simulink model "mfordmodel_v1"  (R2023a)
settings: Solver=ode45  StartTime=0.0  StopTime=10.0  RelTol=1e-3  EnableMultiTasking=on
undefined symbols (not defined in the file): ABV_RATIO_SW, AC_OFF_DLY, ACLOD, AUTO_TRNS_SW, BRAKE_DNDT_X, BZZRPM, BZZRPM_ALT, BZZTM, BZZTM_ALT, CMD_LITOFF, CMD_STABLE, CO_ST_ECT__A, COOL_BASE, DAS_BKDLY_A, DAS_CNT, DAS_CTDLY, DAS_LC_SW__A, DASCLP_5INH, DASCTL, DASMHYST, DASMPH, DEBYCP, DES_BASE, DPNEU_MUL, DSDRPM_DN_TC, DSDRPM_OFF, DSDRPM_UP_TC, EDF_DELAY, EDFHP, ETC_CL_TP, ETC_HP, GR_CM_CREEP, HCAM_ACT_CLP, HEDFHP, HEDFRPM, HICAM_PS, IAC_CAL_SW, IAC_ER_TM1, IAC_ER_TM2, IAC_ER_TM4, IAC_HI_LIM__A, IAC_ISFL_OBD, IAC_KAM_SW, IAC_LO_LIM__A, IAC_MON_TM, IAC_OT_REQ, IAC_RUN_TM, IAC_TP_OBD, IAC_TR_DAS, IAC_TST_DC, ID_DAS__A, ID_NOVS__A, IDVS_CH__A, IDVS_SL__A, IPSI_SW, IPSIDLY, IS_DRBASE__A, IS_DRBASE_A__A, IS_NUBASE__A, IS_NUBASE_A__A ... (+35)
libraries: simulink x2
(part 11 of 12)

== stateflow chart mfordmodel_v1/iac_v04_001_001/iac_executive/misc_calcs/TIMER_DT_in/Timer Control ==
  state TIMER_control
    state CHANGE_timer
      /* only one
      flag active */
      CHANGE_timer -> (junction 25) [order 1]
      (junction 26) -> (junction 25) [order 2]
      (junction 25) -> (junction 28) [order 1] : [incr_flag==1]
          | {
          | count_direction=1;
          | }
      (junction 25) -> (junction 28) [order 2] : [decr_flag==1]
          | {
          | count_direction= -1;
          | }
      (default) -> (junction 26)
      (junction 26) -> (junction 30) [order 1] : [reset_flag == 1]
          | {reset_flag = 0;}
      (junction 28) -> (junction 30) : {
          | do_delta_time;
          | do_timer;
          | }
    state HOLD_timer
      /* flags both
      active or both
      inactive */
      (default) -> (junction 27)
      (junction 27) -> (junction 29) : {
          | count_direction=0;
          | do_delta_time;
          | }
    (default) -> (junction 23)
    (junction 23) -> HOLD_timer [order 2]
    (junction 23) -> CHANGE_timer [order 1] : [incr_flag!=decr_flag]
    HOLD_timer -> (junction 27) [order 2]
    HOLD_timer -> CHANGE_timer [order 1] : [incr_flag!=decr_flag]
    CHANGE_timer -> HOLD_timer [order 1] : [incr_flag==decr_flag]
  (default) -> (junction 24)
  (junction 24) -> TIMER_control [order 2]
  (junction 24) -> TIMER_control [order 1] : trig_reset
      | {
      | reset_flag=1;
      | do_delta_time;
      | do_timer;
      | }
  TIMER_control -> TIMER_control : trig_reset
      | {
      | reset_flag=1;
      | do_delta_time;
      | do_timer;
      | }
  data: count_direction output int16; incr_flag input boolean; decr_flag input boolean; reset_flag output boolean [0..1]
  events: do_delta_time output FUNCTION_CALL_EVENT; do_timer output FUNCTION_CALL_EVENT; trig_timer input FUNCTION_CALL_EVENT; trig_reset input FUNCTION_CALL_EVENT

== stateflow chart mfordmodel_v1/iac_v04_001_001/activate_desired_rpm/rpm_adders_fans_and_pw_steer/rpm_adders_fans_pw_steer_ctl ==
  (default) -> (junction 6) : trig_rpm_adders_fans_pw_steer
  (junction 6) -> (junction 7) [order 2] : { is_hedf_rpm = 0.0; }
  (junction 6) -> (junction 7) [order 1] : [   (HEDFHP == 1)...
      |  && (hsf_flg == 1) ]
      | { is_hedf_rpm =HEDFRPM; }
  (junction 7) -> (junction 8) [order 1] : [ powsfg == 1 ]
      | { is_ps_rpm = PS_RPM; }
  (junction 7) -> (junction 8) [order 2] : { is_ps_rpm = 0.0; }
  data: HEDFHP parameter boolean size=1; hsf_flg input boolean size=1; is_hedf_rpm output double size=1; powsfg input boolean size=1; is_ps_rpm output double size=1; PS_RPM parameter double size=1; HEDFRPM parameter double size=1
  events: trig_rpm_adders_fans_pw_steer input FUNCTION_CALL_EVENT

== stateflow chart mfordmodel_v1/iac_v04_001_001/iac_executive/runup_flag_timer/TIMER_DT_in/Timer Control ==
  state TIMER_control
    state CHANGE_timer
      /* only one
      flag active */
      CHANGE_timer -> (junction 25) [order 1]
      (junction 26) -> (junction 25) [order 2]
      (junction 25) -> (junction 28) [order 1] : [incr_flag==1]
          | {
          | count_direction=1;
          | }
      (junction 25) -> (junction 28) [order 2] : [decr_flag==1]
          | {
          | count_direction= -1;
          | }
      (default) -> (junction 26)
      (junction 26) -> (junction 30) [order 1] : [reset_flag == 1]
          | {reset_flag = 0;}
      (junction 28) -> (junction 30) : {
          | do_delta_time;
          | do_timer;
          | }
    state HOLD_timer
      /* flags both
      active or both
      inactive */
      (default) -> (junction 27)
      (junction 27) -> (junction 29) : {
          | count_direction=0;
          | do_delta_time;
          | }
    (default) -> (junction 23)
    (junction 23) -> HOLD_timer [order 2]
    (junction 23) -> CHANGE_timer [order 1] : [incr_flag!=decr_flag]
    HOLD_timer -> (junction 27) [order 2]
    HOLD_timer -> CHANGE_timer [order 1] : [incr_flag!=decr_flag]
    CHANGE_timer -> HOLD_timer [order 1] : [incr_flag==decr_flag]
  (default) -> (junction 24)
  (junction 24) -> TIMER_control [order 2]
  (junction 24) -> TIMER_control [order 1] : trig_reset
      | {
      | reset_flag=1;
      | do_delta_time;
      | do_timer;
      | }
  TIMER_control -> TIMER_control : trig_reset
      | {
      | reset_flag=1;
      | do_delta_time;
      | do_timer;
      | }
  data: count_direction output int16; incr_flag input boolean; decr_flag input boolean; reset_flag output boolean [0..1]
  events: do_delta_time output FUNCTION_CALL_EVENT; do_timer output FUNCTION_CALL_EVENT; trig_timer input FUNCTION_CALL_EVENT; trig_reset input FUNCTION_CALL_EVENT

== stateflow chart mfordmodel_v1/iac_v04_001_001/normal_mode/activate_feedforward/ac_ppm_tmr/Timer Control ==
  state TIMER_control
    state CHANGE_timer
      /* only one
      flag active */
      CHANGE_timer -> (junction 23) [order 1]
      (default) -> (junction 23)
      (junction 23) -> (junction 25) [order 1] : [incr_flag==1]
          | {
          | count_direction=1;
          | }
      (junction 23) -> (junction 25) [order 2] : [decr_flag==1]
          | {
          | count_direction=(-1);
          | }
      (junction 25) -> (junction 27) : {
          | do_delta_time;
          | do_timer;
          | }
    state HOLD_timer
      /* flags both
      active or both
      inactive */
      (default) -> (junction 24)
      (junction 24) -> (junction 26) : {
          | count_direction=0;
          | do_delta_time;
          | }
    (default) -> (junction 21) : {
        | reset_flag=0;
        | }
    (junction 21) -> HOLD_timer [order 2]
    (junction 21) -> CHANGE_timer [order 1] : [incr_flag!=decr_flag]
    HOLD_timer -> (junction 24) [order 2]
    HOLD_timer -> CHANGE_timer [order 1] : [incr_flag!=decr_flag]
    CHANGE_timer -> HOLD_timer [order 1] : [incr_flag==decr_flag]
  (default) -> (junction 22)
  (junction 22) -> TIMER_control [order 2]
  (junction 22) -> TIMER_control [order 1] : trig_reset
      | {
      | reset_flag=1;
      | do_delta_time;
      | do_timer;
      | }
  TIMER_control -> TIMER_control : trig_reset
      | {
      | reset_flag=1;
      | do_delta_time;
      | do_timer;
      | }
  data: count_direction output int16; incr_flag input boolean; decr_flag input boolean; reset_flag output boolean [0..1]
  events: do_delta_time output FUNCTION_CALL_EVENT; do_timer output FUNCTION_CALL_EVENT; trig_timer input FUNCTION_CALL_EVENT; trig_reset input FUNCTION_CALL_EVENT

== stateflow chart mfordmodel_v1/iac_v04_001_001/normal_mode/activate_kam/iac_kam_tmr/Timer Control ==
  state TIMER_control
    state CHANGE_timer
      /* only one
      flag active */
      CHANGE_timer -> (junction 23) [order 1]
      (default) -> (junction 23)
      (junction 23) -> (junction 25) [order 1] : [incr_flag==1]
          | {
          | count_direction=1;
          | }
      (junction 23) -> (junction 25) [order 2] : [decr_flag==1]
          | {
          | count_direction=(-1);
          | }
      (junction 25) -> (junction 27) : {
          | do_delta_time;
          | do_timer;
          | }
    state HOLD_timer
      /* flags both
      active or both
      inactive */
      (default) -> (junction 24)
      (junction 24) -> (junction 26) : {
          | count_direction=0;
          | do_delta_time;
          | }
    (default) -> (junction 21) : {
        | reset_flag=0;
        | }
    (junction 21) -> HOLD_timer [order 2]
    (junction 21) -> CHANGE_timer [order 1] : [incr_flag!=decr_flag]
    HOLD_timer -> (junction 24) [order 2]
    HOLD_timer -> CHANGE_timer [order 1] : [incr_flag!=decr_flag]
    CHANGE_timer -> HOLD_timer [order 1] : [incr_flag==decr_flag]
  (default) -> (junction 22)
  (junction 22) -> TIMER_control [order 2]
  (junction 22) -> TIMER_control [order 1] : trig_reset
      | {
      | reset_flag=1;
      | do_delta_time;
      | do_timer;
      | }
  TIMER_control -> TIMER_control : trig_reset
      | {
      | reset_flag=1;
      | do_delta_time;
      | do_timer;
      | }
  data: count_direction output int16; incr_flag input boolean; decr_flag input boolean; reset_flag output boolean [0..1]
  events: do_delta_time output FUNCTION_CALL_EVENT; do_timer output FUNCTION_CALL_EVENT; trig_timer input FUNCTION_CALL_EVENT; trig_reset input FUNCTION_CALL_EVENT

== stateflow chart mfordmodel_v1/iac_v04_001_001/normal_mode/activate_normal_mode/normal_mode_fault_codes/iac_er_tmr1/Timer Control ==
  state TIMER_control
    state CHANGE_timer
      /* only one
      flag active */
      CHANGE_timer -> (junction 23) [order 1]
      (default) -> (junction 23)
      (junction 23) -> (junction 25) [order 1] : [incr_flag==1]
          | {
          | count_direction=1;
          | }
      (junction 23) -> (junction 25) [order 2] : [decr_flag==1]
          | {
          | count_direction=(-1);
          | }
      (junction 25) -> (junction 27) : {
          | do_delta_time;
          | do_timer;
          | }
    state HOLD_timer
      /* flags both
      active or both
      inactive */
      (default) -> (junction 24)
      (junction 24) -> (junction 26) : {
          | count_direction=0;
          | do_delta_time;
          | }
    (default) -> (junction 21) : {
        | reset_flag=0;
        | }
    (junction 21) -> HOLD_timer [order 2]
    (junction 21) -> CHANGE_timer [order 1] : [incr_flag!=decr_flag]
    HOLD_timer -> (junction 24) [order 2]
    HOLD_timer -> CHANGE_timer [order 1] : [incr_flag!=decr_flag]
    CHANGE_timer -> HOLD_timer [order 1] : [incr_flag==decr_flag]
  (default) -> (junction 22)
  (junction 22) -> TIMER_control [order 2]
  (junction 22) -> TIMER_control [order 1] : trig_reset
      | {
      | reset_flag=1;
      | do_delta_time;
      | do_timer;
      | }
  TIMER_control -> TIMER_control : trig_reset
      | {
      | reset_flag=1;
      | do_delta_time;
      | do_timer;
      | }
  data: count_direction output int16; incr_flag input boolean; decr_flag input boolean; reset_flag output boolean [0..1]
  events: do_delta_time output FUNCTION_CALL_EVENT; do_timer output FUNCTION_CALL_EVENT; trig_timer input FUNCTION_CALL_EVENT; trig_reset input FUNCTION_CALL_EVENT

== stateflow chart mfordmodel_v1/iac_v04_001_001/normal_mode/activate_normal_mode/normal_mode_fault_codes/iac_er_tmr2/Timer Control ==
  state TIMER_control
    state CHANGE_timer
      /* only one
      flag active */
      CHANGE_timer -> (junction 23) [order 1]
      (default) -> (junction 23)
      (junction 23) -> (junction 25) [order 1] : [incr_flag==1]
          | {
          | count_direction=1;
          | }
      (junction 23) -> (junction 25) [order 2] : [decr_flag==1]
          | {
          | count_direction=(-1);
          | }
      (junction 25) -> (junction 27) : {
          | do_delta_time;
          | do_timer;
          | }
    state HOLD_timer
      /* flags both
      active or both
      inactive */
      (default) -> (junction 24)
      (junction 24) -> (junction 26) : {
          | count_direction=0;
          | do_delta_time;
          | }
    (default) -> (junction 21) : {
        | reset_flag=0;
        | }
    (junction 21) -> HOLD_timer [order 2]
    (junction 21) -> CHANGE_timer [order 1] : [incr_flag!=decr_flag]
    HOLD_timer -> (junction 24) [order 2]
    HOLD_timer -> CHANGE_timer [order 1] : [incr_flag!=decr_flag]
    CHANGE_timer -> HOLD_timer [order 1] : [incr_flag==decr_flag]
  (default) -> (junction 22)
  (junction 22) -> TIMER_control [order 2]
  (junction 22) -> TIMER_control [order 1] : trig_reset
      | {
      | reset_flag=1;
      | do_delta_time;
      | do_timer;
      | }
  TIMER_control -> TIMER_control : trig_reset
      | {
      | reset_flag=1;
      | do_delta_time;
      | do_timer;
      | }
  data: count_direction output int16; incr_flag input boolean; decr_flag input boolean; reset_flag output boolean [0..1]
  events: do_delta_time output FUNCTION_CALL_EVENT; do_timer output FUNCTION_CALL_EVENT; trig_timer input FUNCTION_CALL_EVENT; trig_reset input FUNCTION_CALL_EVENT

== stateflow chart mfordmodel_v1/iac_v04_001_001/normal_mode/activate_normal_mode/normal_mode_fault_codes/iac_mon_tmr/Timer Control ==
  state TIMER_control
    state CHANGE_timer
      /* only one
      flag active */
      CHANGE_timer -> (junction 23) [order 1]
      (default) -> (junction 23)
      (junction 23) -> (junction 25) [order 1] : [incr_flag==1]
          | {
          | count_direction=1;
          | }
      (junction 23) -> (junction 25) [order 2] : [decr_flag==1]
          | {
          | count_direction=(-1);
          | }
      (junction 25) -> (junction 27) : {
          | do_delta_time;
          | do_timer;
          | }
    state HOLD_timer
      /* flags both
      active or both
      inactive */
      (default) -> (junction 24)
      (junction 24) -> (junction 26) : {
          | count_direction=0;
          | do_delta_time;
          | }
    (default) -> (junction 21) : {
        | reset_flag=0;
        | }
    (junction 21) -> HOLD_timer [order 2]
    (junction 21) -> CHANGE_timer [order 1] : [incr_flag!=decr_flag]
    HOLD_timer -> (junction 24) [order 2]
    HOLD_timer -> CHANGE_timer [order 1] : [incr_flag!=decr_flag]
    CHANGE_timer -> HOLD_timer [order 1] : [incr_flag==decr_flag]
  (default) -> (junction 22)
  (junction 22) -> TIMER_control [order 2]
  (junction 22) -> TIMER_control [order 1] : trig_reset
      | {
      | reset_flag=1;
      | do_delta_time;
      | do_timer;
      | }
  TIMER_control -> TIMER_control : trig_reset
      | {
      | reset_flag=1;
      | do_delta_time;
      | do_timer;
      | }
  data: count_direction output int16; incr_flag input boolean; decr_flag input boolean; reset_flag output boolean [0..1]
  events: do_delta_time output FUNCTION_CALL_EVENT; do_timer output FUNCTION_CALL_EVENT; trig_timer input FUNCTION_CALL_EVENT; trig_reset input FUNCTION_CALL_EVENT

== stateflow chart mfordmodel_v1/iac_v04_001_001/normal_mode/activate_normal_mode/normal_mode_fault_codes/type1_fault_code/fault code_ctl ==
  state clear [parallel]
    settings: executionOrder=1
    clear -> (junction 9) : clear_malf
    (default) -> (junction 9) : clear_malf
    (junction 9) -> (junction 12) : {pxxxmalf = 0;}
  state malf [parallel]
    settings: executionOrder=2
    malf -> (junction 10) : malfunction
    (default) -> (junction 10) : malfunction
    (junction 10) -> (junction 11) : {pxxxmalf = 1;}
  data: pxxxmalf output double
  events: malfunction input FUNCTION_CALL_EVENT; clear_malf input FUNCTION_CALL_EVENT

== stateflow chart mfordmodel_v1/iac_v04_001_001/normal_mode/activate_normal_mode/normal_mode_fault_codes/type1_fault_code1/fault code_ctl ==
  state clear [parallel]
    settings: executionOrder=1
    clear -> (junction 9) : clear_malf
    (default) -> (junction 9) : clear_malf
    (junction 9) -> (junction 12) : {pxxxmalf = 0;}
  state malf [parallel]
    settings: executionOrder=2
    malf -> (junction 10) : malfunction
    (default) -> (junction 10) : malfunction
    (junction 10) -> (junction 11) : {pxxxmalf = 1;}
  data: pxxxmalf output double
  events: malfunction input FUNCTION_CALL_EVENT; clear_malf input FUNCTION_CALL_EVENT

== stateflow chart mfordmodel_v1/iac_v04_001_001/normal_mode/iscflg_module/dashpot/TIMER/Timer Control ==
  state TIMER_control
    state CHANGE_timer
      /* only one
      flag active */
      CHANGE_timer -> (junction 23) [order 1]
      (default) -> (junction 23)
      (junction 23) -> (junction 25) [order 1] : [incr_flag==1]
          | {
          | count_direction=1;
          | }
      (junction 23) -> (junction 25) [order 2] : [decr_flag==1]
          | {
          | count_direction=(-1);
          | }
      (junction 25) -> (junction 27) : {
          | do_delta_time;
          | do_timer;
          | }
    state HOLD_timer
      /* flags both
      active or both
      inactive */
      (default) -> (junction 24)
      (junction 24) -> (junction 26) : {
          | count_direction=0;
          | do_delta_time;
          | }
    (default) -> (junction 21) : {
        | reset_flag=0;
        | }
    (junction 21) -> HOLD_timer [order 2]
    (junction 21) -> CHANGE_timer [order 1] : [incr_flag!=decr_flag]
    HOLD_timer -> (junction 24) [order 2]
    HOLD_timer -> CHANGE_timer [order 1] : [incr_flag!=decr_flag]
    CHANGE_timer -> HOLD_timer [order 1] : [incr_flag==decr_flag]
  (default) -> (junction 22)
  (junction 22) -> TIMER_control [order 2]
  (junction 22) -> TIMER_control [order 1] : trig_reset
      | {
      | reset_flag=1;
      | do_delta_time;
      | do_timer;
      | }
  TIMER_control -> TIMER_control : trig_reset
      | {
      | reset_flag=1;
      | do_delta_time;
      | do_timer;
      | }
  data: count_direction output int16; incr_flag input boolean; decr_flag input boolean; reset_flag output boolean [0..1]
  events: do_delta_time output FUNCTION_CALL_EVENT; do_timer output FUNCTION_CALL_EVENT; trig_timer input FUNCTION_CALL_EVENT; trig_reset input FUNCTION_CALL_EVENT

== stateflow chart mfordmodel_v1/iac_v04_001_001/normal_mode/iscflg_module/iscflg_modes/1/Timer Control ==
  state TIMER_control
    state CHANGE_timer
      /* only one
      flag active */
      CHANGE_timer -> (junction 23) [order 1]
      (default) -> (junction 23)
      (junction 23) -> (junction 25) [order 1] : [incr_flag==1]
          | {
          | count_direction=1;
          | }
      (junction 23) -> (junction 25) [order 2] : [decr_flag==1]
          | {
          | count_direction=(-1);
          | }
      (junction 25) -> (junction 27) : {
          | do_delta_time;
          | do_timer;
          | }
    state HOLD_timer
      /* flags both
      active or both
      inactive */
      (default) -> (junction 24)
      (junction 24) -> (junction 26) : {
          | count_direction=0;
          | do_delta_time;
          | }
    (default) -> (junction 21) : {
        | reset_flag=0;
        | }
    (junction 21) -> HOLD_timer [order 2]
    (junction 21) -> CHANGE_timer [order 1] : [incr_flag!=decr_flag]
    HOLD_timer -> (junction 24) [order 2]
    HOLD_timer -> CHANGE_timer [order 1] : [incr_flag!=decr_flag]
    CHANGE_timer -> HOLD_timer [order 1] : [incr_flag==decr_flag]
  (default) -> (junction 22)
  (junction 22) -> TIMER_control [order 2]
  (junction 22) -> TIMER_control [order 1] : trig_reset
      | {
      | reset_flag=1;
      | do_delta_time;
      | do_timer;
      | }
  TIMER_control -> TIMER_control : trig_reset
      | {
      | reset_flag=1;
      | do_delta_time;
      | do_timer;
      | }
  data: count_direction output int16; incr_flag input boolean; decr_flag input boolean; reset_flag output boolean [0..1]
  events: do_delta_time output FUNCTION_CALL_EVENT; do_timer output FUNCTION_CALL_EVENT; trig_timer input FUNCTION_CALL_EVENT; trig_reset input FUNCTION_CALL_EVENT

== stateflow chart mfordmodel_v1/iac_v04_001_001/iac_executive/misc_calcs/misc_calcs_ctl ==
  (default) -> (junction 9) : {
      |  trig_osc_response_logic;
      | }
  (junction 9) -> (junction 11) [order 2] : /* gear5tmr_update */
  (junction 9) -> (junction 10) [order 1] : [ TRLOAD > 3 ]
  (junction 10) -> (junction 11) [order 1] : [ gr_cm != 5 ]
      | {
      |   gear5th = 0;
      |   trig_rst_gear5tmr;
      | }
  (junction 10) -> (junction 11) [order 2] : {
      |  gear5th = 1;
      |  trig_incr_gear5tmr;
      | }
  (junction 11) -> (junction 12) [order 1] : /* dndt_das_update() */
      |
      | [  (eng_stalled == 1)...
      |  || ( apt >= 0) ]
      | {
      | ml_dndt_sw = 1;
      | }
  (junction 11) -> (junction 12) [order 2] : {
      |  ml_dndt_sw = 2;
      | }
  (junction 12) -> (junction 13) : {
      | do_dndt_calc;
      | }
  data: TRLOAD parameter uint8 size=1; gear5th output boolean size=1; ml_dndt_sw output uint8 size=1 =1; eng_stalled input boolean size=1; gr_cm input uint8 size=1; apt input int8 size=1
  events: trig_incr_gear5tmr output FUNCTION_CALL_EVENT; trig_rst_gear5tmr output FUNCTION_CALL_EVENT; trig_misc_calcs input FUNCTION_CALL_EVENT; do_dndt_calc output FUNCTION_CALL_EVENT; trig_osc_response_logic output FUNCTION_CALL_EVENT

== stateflow chart mfordmodel_v1/iac_v04_001_001/normal_mode/iscflg_module/iscflg_modes/2/Timer Control ==
  state TIMER_control
    state CHANGE_timer
      /* only one
      flag active */
      CHANGE_timer -> (junction 23) [order 1]
      (default) -> (junction 23)
      (junction 23) -> (junction 25) [order 1] : [incr_flag==1]
          | {
          | count_direction=1;
          | }
      (junction 23) -> (junction 25) [order 2] : [decr_flag==1]
          | {
          | count_direction=(-1);
          | }
      (junction 25) -> (junction 27) : {
          | do_delta_time;
          | do_timer;
          | }
    state HOLD_timer
      /* flags both
      active or both
      inactive */
      (default) -> (junction 24)
      (junction 24) -> (junction 26) : {
          | count_direction=0;
          | do_delta_time;
          | }
    (default) -> (junction 21) : {
        | reset_flag=0;
        | }
    (junction 21) -> HOLD_timer [order 2]
    (junction 21) -> CHANGE_timer [order 1] : [incr_flag!=decr_flag]
    HOLD_timer -> (junction 24) [order 2]
    HOLD_timer -> CHANGE_timer [order 1] : [incr_flag!=decr_flag]
    CHANGE_timer -> HOLD_timer [order 1] : [incr_flag==decr_flag]
  (default) -> (junction 22)
  (junction 22) -> TIMER_control [order 2]
  (junction 22) -> TIMER_control [order 1] : trig_reset
      | {
      | reset_flag=1;
      | do_delta_time;
      | do_timer;
      | }
  TIMER_control -> TIMER_control : trig_reset
      | {
      | reset_flag=1;
      | do_delta_time;
      | do_timer;
      | }
  data: count_direction output int16; incr_flag input boolean; decr_flag input boolean; reset_flag output boolean [0..1]
  events: do_delta_time output FUNCTION_CALL_EVENT; do_timer output FUNCTION_CALL_EVENT; trig_timer input FUNCTION_CALL_EVENT; trig_reset input FUNCTION_CALL_EVENT

== stateflow chart mfordmodel_v1/iac_v04_001_001/normal_mode/activate_feedforward/activate_feedforward_ctl ==
  state ac_ppm [parallel]
    settings: executionOrder=1
    ac_ppm -> (junction 43) : trig
    (default) -> (junction 43) : trig
    (junction 43) -> (junction 47) [order 1] : [ ac_ppm_rqst == 0 ]
        | {
        | ml_ac_sw = 3 ;
        | }
    (junction 43) -> (junction 45) [order 2]
    (junction 45) -> (junction 47) [order 2] : {
        | ml_ac_sw = 1 ;
        | }
    (junction 45) -> (junction 47) [order 1] : [ ac_cycle_flg == 0 ]
        | {
        | ml_ac_sw = 2 ;
        | }
    (junction 47) -> (junction 49) [order 2] : {
        | trig_ac_ppm_tmr_update;
        | }
    (junction 47) -> (junction 49) [order 1] : [ ac_ppm_rqst == 0 ]
        | {
        | trig_ac_ppm_tmr_reset;
        | }
  state fan_ppm_calc [parallel]
    settings: executionOrder=2
    fan_ppm_calc -> (junction 42) : trig
    (junction 42) -> (junction 48) [order 1] : [ (EDFHP == 1)...
        |  && ( VSFOP_HP== 0 )...
        |  && (VFD_HP == 0 )...
        |  && ( lsf_rqst == 1 )...
        |  && ( fantmr >= EDF_DELAY) ]
        | {
        | ml_fan_sw = 1;
        | }
    (default) -> (junction 42) : trig
    (junction 42) -> (junction 44) [order 2]
    (junction 44) -> (junction 48) [order 1] : [ VSFOP_HP == 1 ]
        | {
        | ml_fan_sw = 2;
        | }
    (junction 44) -> (junction 46) [order 2]
    (junction 46) -> (junction 48) [order 2] : {
        | ml_fan_sw = 4;
        | }
    (junction 46) -> (junction 48) [order 1] : [ VFD_HP == 1 ]
        | {
        | ml_fan_sw = 3;
        | }
  state base_ppm [parallel]
    settings: executionOrder=3
    base_ppm -> (junction 50) : trig
    (default) -> (junction 50) : trig
    (junction 50) -> (junction 52) [order 1] : [ (AUTO_TRNS_SW == 0 )...
        |  || ( dndsup == 0 ) ]
        | {
        | ml_base_sw = 1  ;
        | }
    (junction 50) -> (junction 52) [order 2] : {
        | ml_base_sw = 2 ;
        | }
    (junction 52) -> (junction 55) [order 2] : {
        | ml_trans_sw = 2 ;
        | }
    (junction 52) -> (junction 55) [order 1] : [  ( idle_ppm <= DASCTL )...
        |  && (      ( pdl != PARK)...
        |          && (pdl != NEUTRAL) )...
        |  && ( apt == CLOSED_THROTTLE )...
        |  && ( ect > VSEECT )...
        |  && ( DES_BASE == 1 )...
        |  && ( vspd > MINMPH )...
        |  && ( gr_cm >= GR_CM_CREEP ) ]
        | {
        | ml_trans_sw = 1;
        | }
  state power_steering_ppm [parallel]
    settings: executionOrder=4
    power_steering_ppm -> (junction 51) : trig
    (default) -> (junction 51) : trig
    (junction 51) -> (junction 53) [order 1] : [  (powsfg == 1)...
        |  && ( PSPSHP == 1)...
        |  && ( hicam <= HICAM_PS) ]
    (junction 51) -> (junction 54) [order 2] : {
        | ml_ps_sw = 3;
        | }
    (junction 53) -> (junction 54) [order 2] : {
        | ml_ps_sw = 2 ;
        | }
    (junction 53) -> (junction 54) [order 1] : [ vspd < PS_VS ]
        | {
        | ml_ps_sw = 1 ;
        | }
  state fail_safe_cooling_ppm [parallel]
    settings: executionOrder=5
    fail_safe_cooling_ppm -> (junction 56) : trig
    (default) -> (junction 56) : trig
    (junction 56) -> (junction 58) [order 2] : {
        | ml_fsc_sw = 2 ;
        | }
    (junction 56) -> (junction 58) [order 1] : [ cool_flg == 1 ]
        | {
        | ml_fsc_sw = 1 ;
        | }
  state desmaf_pre_calcs [parallel]
    /* Must be lowest priority parallel state */
    settings: executionOrder=6
    desmaf_pre_calcs -> (junction 57) : trig_activate_feedforward
    (default) -> (junction 57) : trig_activate_feedforward
    (junction 57) -> (junction 59) : {
        | ac_ppm.trig;
        | fail_safe_cooling_ppm.trig;
        | fan_ppm_calc.trig;
        | base_ppm.trig;
        | power_steering_ppm.trig;
        | do_desmaf_pre_calc;
        | }
  data: dndsup input boolean size=1; ect input single size=1; idle_ppm input single size=1; pdl input uint8 size=1; apt input int8 size=1; vspd input single size=1; gr_cm input uint8 size=1; AUTO_TRNS_SW parameter uint8 size=1; DASCTL parameter single size=1; MINMPH parameter single size=1; VSEECT parameter single size=1; DES_BASE parameter single size=1; ac_cycle_flg input boolean size=1; ac_ppm_rqst input boolean size=1; ml_ac_sw output uint8 size=1; PS_VS parameter single size=1; PSPSHP parameter boolean size=1; powsfg input boolean size=1; cool_flg input boolean size=1; ml_ps_sw output uint8 size=1; ml_fsc_sw output uint8 size=1; ml_base_sw output uint8 size=1; ml_trans_sw output uint8 size=1; hicam input single size=1; HICAM_PS parameter single size=1; AUTOMATIC4 constant uint8 size=1 =4; CLOSED_THROTTLE constant int8 size=1 =-1; ml_fan_sw output int8 size=1 =3; VSFOP_HP parameter boolean size=1; EDFHP parameter boolean size=1; lsf_rqst input boolean size=1; EDF_DELAY parameter single size=1; fantmr input single size=1; VFD_HP parameter single size=1; GR_CM_CREEP parameter uint8 size=1; PARK constant uint8 size=1 =70; NEUTRAL constant uint8 size=1 =50
  events: trig local EITHER_EDGE_EVENT; trig local EITHER_EDGE_EVENT; trig local EITHER_EDGE_EVENT; trig local EITHER_EDGE_EVENT; trig local EITHER_EDGE_EVENT; trig_activate_feedforward input FUNCTION_CALL_EVENT; do_desmaf_pre_calc output FUNCTION_CALL_EVENT; trig_ac_ppm_tmr_update output FUNCTION_CALL_EVENT; trig_ac_ppm_tmr_reset output FUNCTION_CALL_EVENT

== stateflow chart mfordmodel_v1/iac_v04_001_001/normal_mode/iscflg_module/dashpot/activate_daspot_mode_ctl ==
  (default) -> (junction 20) : { trig_dec_das_delay; }
  (junction 20) -> (junction 21) [order 1] : /* no_decel_counter() */
      | [ ( gear5th == 0) ||...
      |   ( cttmr <= DAS_CTDLY) ]
  (junction 21) -> (junction 26) : { das_ctr = 0; }
  (junction 20) -> (junction 22) [order 2]
  (junction 22) -> (junction 23) [order 1] : [ (gear5th == 1) &&...
      |   ( cttmr > DAS_CTDLY) &&...
      |   ( dndt_das > DAS_DNDT_X) &&...
      |   ( das_ctr < 255 ) ]
  (junction 23) -> (junction 25) : { das_ctr = das_ctr + 1; }
  (junction 22) -> (junction 24) [order 2]
  (junction 25) -> (junction 24)
  (junction 26) -> (junction 25)
  (junction 24) -> (junction 27) : { trig_daspot_shift_trans_calc; }
  (junction 27) -> (junction 28) [order 1] : /* base_dashpot_calculation() */
      | [ (das_delay__A > 0.0)...
      |  && (das_ppm__A > 0.0) ]
  (junction 28) -> (junction 32) : { ml_idle_ppm_sw = 1; }
  (junction 27) -> (junction 29) [order 2]
  (junction 29) -> (junction 30) [order 1] : [ (flg_crv_lk == 1)...
      |  && (DAS_LC_SW__A == 1) ]
  (junction 30) -> (junction 33) : { ml_idle_ppm_sw = 2; }
  (junction 29) -> (junction 31) [order 2] : { ml_idle_ppm_sw = 3; }
  (junction 33) -> (junction 31)
  (junction 32) -> (junction 33)
  (junction 31) -> (junction 34) : { do_daspot_calc;
      |   trig_das_min_clip_daspot; }
  data: ml_idle_ppm_sw output uint8 size=1; das_delay__A input double size=1; das_ppm__A input double size=1; gear5th input boolean size=1; cttmr input single size=1; DAS_CTDLY parameter single size=1; DAS_DNDT_X constant single size=1; das_ctr output uint8 size=1; dndt_das input single size=1; ndsflg input boolean size=1; ptctfg input boolean size=1; TRLOAD parameter uint8 size=1; NRATCH_OFF constant boolean size=1; DAS_LC_SW__A constant boolean size=1; flg_crv_lk input boolean size=1; engine_speed input single size=1; CLOSED_THROTTLE constant int8 size=1 =-1; apt input int8 size=1
  events: trig_activate_daspot_mode input FUNCTION_CALL_EVENT; do_daspot_calc output FUNCTION_CALL_EVENT; trig_das_min_clip_daspot output FUNCTION_CALL_EVENT; trig_dec_das_delay output FUNCTION_CALL_EVENT; trig_daspot_shift_trans_calc output FUNCTION_CALL_EVENT

== stateflow chart mfordmodel_v1/iac_v04_001_001/normal_mode/iscflg_module/das_min_clip/das_min_clip_ctl ==
  state min_clip_calc [parallel]
    settings: executionOrder=1
    (default) -> (junction 88) : trig
    min_clip_calc -> (junction 88) : trig
    (junction 88) -> (junction 89) [order 1] : [ (dndsup == 0) && (TRLOAD > 3) ]
    (junction 89) -> (junction 91)
    (junction 88) -> (junction 90) [order 2]
    (junction 90) -> (junction 91) [order 1] : [ (DASCLP_5INH == 1) && (apt >= 0) && (gear5th == 1) && (flg_dasclp5 == 0) ]
    (junction 91) -> (junction 93)
    (junction 90) -> (junction 92) [order 2]
    (junction 92) -> (junction 93) [order 1] : [ (gear5tmr > DAS_BKDLY_A) && (dndt_das < BRAKE_DNDT_X) ]
    (junction 93) -> (junction 95)
    (junction 92) -> (junction 94) [order 2]
    (junction 94) -> (junction 95) [order 1] : [ (tfmflg == 1) || (flg_dasmnq == 0) ]
    (junction 95) -> (junction 107) : { das_min_clp = 0.0;
        |   das_clp_st = 0; }
    (junction 94) -> (junction 96) [order 2]
    (junction 96) -> (junction 97) [order 1] : [ (TRLOAD > 3) && ( gear5th == 0) ]
    (junction 97) -> (junction 101)
    (junction 96) -> (junction 100) [order 2]
    (junction 100) -> (junction 101) [order 1] : [ (TRLOAD <= 3) && (dndsup == 1) ]
    (junction 101) -> (junction 106) : { das_min_clp = ml_fn894;
        |   das_clp_st = 1; }
    (junction 100) -> (junction 104) [order 2]
    (junction 104) -> (junction 105) [order 1] : [ TRLOAD <= 3 ]
    (junction 106) -> (junction 107)
    (junction 105) -> (junction 111) : { das_min_clp = ( ml_fn894 * DPNEU_MUL );
        |   das_clp_st = 2; }
    (junction 107) -> (junction 112)
    (junction 104) -> (junction 115) [order 2]
    (junction 111) -> (junction 112)
    (junction 112) -> (junction 123)
    (junction 115) -> (junction 114) [order 1] : [ ( das_ctr >= DAS_CNT) &&...
        |   ( flg_crv_lk == 1 ) &&...
        |   ( DAS_LC_SW__A == 1) ]
    (junction 114) -> (junction 116) [order 1] : [ das_clp_st >= 3]
    (junction 116) -> (junction 120) : { das_min_clp = ml_rolav_llc; }
    (junction 115) -> (junction 125) [order 2]
    (junction 114) -> (junction 119) [order 2] : { das_min_clp = ml_fn894llc; }
    (junction 119) -> (junction 120)
    (junction 120) -> (junction 122) : { dasl_min_clp = ml_fn894llc;
        |   das_clp_st = 3; }
    (junction 122) -> (junction 123)
    (junction 123) -> (junction 128)
    (junction 125) -> (junction 126) [order 1] : [ ( das_ctr >= DAS_CNT ) && ...
        |   ( das_clp_st >= 3 ) &&...
        |   ( DAS_LC_SW__A == 1) ]
    (junction 126) -> (junction 127) : { das_min_clp = ml_rolav_l;
        |    das_clp_st = 4;
        |    dasl_min_clp = ml_fn894l; }
    (junction 125) -> (junction 129) [order 2]
    (junction 127) -> (junction 128)
    (junction 128) -> (junction 136)
    (junction 129) -> (junction 131) [order 1] : [ das_ctr >= DAS_CNT ]
    (junction 131) -> (junction 135) : { das_min_clp = ml_fn894l
        |    das_clp_st = 4;
        |    dasl_min_clp = ml_fn894l; }
    (junction 129) -> (junction 137) [order 2]
    (junction 135) -> (junction 136)
    (junction 136) -> (junction 140)
    (junction 137) -> (junction 138) [order 1] : [ ( flg_crv_lk == 1 ) &&...
        |    ( das_clp_st >= 3 ) && ...
        |    ( DAS_LC_SW__A == 1 ) ]
    (junction 138) -> (junction 139) : { das_min_clp = ml_rolav_hlc;
        |   das_clp_st = 5;
        |   dasl_min_clp = ml_fn894hlc; }
    (junction 137) -> (junction 141) [order 2]
    (junction 139) -> (junction 140)
    (junction 141) -> (junction 142) [order 1] : [ ( flg_crv_lk == 1 ) &&...
        |   ( DAS_LC_SW__A == 1 ) ]
    (junction 140) -> (junction 144)
    (junction 142) -> (junction 143) : { das_min_clp =  ml_fn894hlc;
        |   das_clp_st = 5;
        |   dasl_min_clp = ml_fn894hlc; }
    (junction 141) -> (junction 145) [order 2]
    (junction 143) -> (junction 144)
    (junction 144) -> (junction 149)
    (junction 145) -> (junction 146) [order 1] : [ (das_clp_st >= 3 ) &&...
        |   (DAS_LC_SW__A == 1) ]
    (junction 146) -> (junction 148) : { das_min_clp = ml_rolav_h;
        |    das_clp_st = 6;
        |    dasl_min_clp = ml_fn894h; }
    (junction 145) -> (junction 147) [order 2] : { das_min_clp  = ml_fn894h;
        |    das_clp_st   = 6
        |    dasl_min_clp = ml_fn894h; }
    (junction 148) -> (junction 147)
    (junction 149) -> (junction 148)
    (junction 147) -> (junction 150)
  state Note: [group]
    Parallel state "das_min_clip" is
    the main entry point and must be set
    to a lower priority than "min_clip_calc"
    for initial execution sequencing.
  state das_min_clp [parallel]
    settings: executionOrder=2
    (default) -> (junction 98)
    das_min_clp -> (junction 98)
    (junction 98) -> (junction 99) [order 1] : [ (engine_speed <= n_ratch )...
        |  && (apt == CLOSED_THROTTLE) ]
    (junction 99) -> (junction 103)
    (junction 98) -> (junction 102) [order 2]
    (junction 102) -> (junction 103) [order 1] : [ (ptctfg == 1) || (NRATCH_OFF == 1) ]
    (junction 103) -> (junction 109)
    (junction 102) -> (junction 108) [order 2]
    (junction 108) -> (junction 109) [order 1] : [ (ndsflg == 1) && (TRLOAD == 3) ]
    (junction 109) -> (junction 113) : { n_ratch = engine_speed; }
    (junction 108) -> (junction 110) [order 2]
    (junction 113) -> (junction 110)
    (junction 110) -> (junction 117) : { do_functions; }
    (junction 117) -> (junction 118) [order 1] : [ (apt >= 0) && (idle_ppm_in >= ml_fn894h) ]
    (junction 118) -> (junction 133) : { flg_dasclp5 = 1; }
    (junction 117) -> (junction 121) [order 2]
    (junction 121) -> (junction 124) [order 1] : [ apt == CLOSED_THROTTLE ]
    (junction 124) -> (junction 132) : { flg_dasclp5 = 0; }
    (junction 121) -> (junction 130) [order 2]
    (junction 132) -> (junction 130)
    (junction 133) -> (junction 132)
    (junction 130) -> (junction 134) : { min_clip_calc.trig; }
  data: dndsup input boolean size=1; das_min_clp output single size=1; engine_speed input single size=1; ptctfg input boolean size=1; ndsflg input single size=1; tfmflg input boolean size=1; apt input int8 size=1; flg_crv_lk input boolean size=1; flg_dasmnq input boolean size=1; gear5tmr input single size=1; das_ctr input uint8 size=1; dndt_das input single size=1; idle_ppm_in input single size=1; gear5th input boolean size=1; ml_fn894hlc input single size=1; ml_fn894llc input single size=1; ml_fn894h input single size=1; ml_fn894l input single size=1; ml_fn894 input single size=1; ml_rolav_h input single size=1; ml_rolav_l input single size=1; ml_rolav_llc input single size=1; ml_rolav_hlc input single size=1; dasl_min_clp output single size=1; n_ratch output single size=1; TRLOAD parameter uint8 size=1; NRATCH_OFF parameter boolean size=1; CLOSED_THROTTLE constant int8 size=1 =-1; DAS_BKDLY_A parameter single size=1; BRAKE_DNDT_X parameter single size=1; DASCLP_5INH parameter uint8 size=1; das_clp_st local uint8 size=1; DAS_CNT parameter uint8 size=1; DPNEU_MUL parameter single size=1; DAS_LC_SW__A parameter boolean size=1; flg_dasclp5 local boolean size=1
  events: trig local EITHER_EDGE_EVENT; do_functions output FUNCTION_CALL_EVENT; trig_das_min_clip_daspot input FUNCTION_CALL_EVENT; trig_das_min_clip_prepos input FUNCTION_CALL_EVENT

== stateflow chart mfordmodel_v1/iac_v04_001_001/normal_mode/iscflg_module/idle_rpm_controller/idle_rpm_controller_ctl ==
  state idle_rpm_controller_initialisation [parallel]
    settings: executionOrder=1
    idle_rpm_controller_initialisation -> (junction 40) : trig
    (default) -> (junction 40) : trig
    (junction 40) -> (junction 43) : {
        |   do_rpmerr_calc;
        |   do_fn852a_calc;
        |   ml_iscpsi_sw = 2;
        |   do_iscpsi_calc;
        |   ml_der_sw = 1;
        |   do_idle_ppm_calc;
        | }
  state normal_rpm_control [parallel]
    settings: executionOrder=2
    normal_rpm_control -> (junction 39) : trig
    (default) -> (junction 39) : trig
    (junction 39) -> (junction 41) : /* Calculate basic error terms */
        | { do_rpmerr_calc; }
    (junction 41) -> (junction 42) [order 2] : { iac_fb_satx = 0; }
    (junction 41) -> (junction 42) [order 1] : [ ipsibr >= PSIBRM ]
        | {  iac_fb_satx = 1; }
    (junction 42) -> (junction 45) [order 1] : [ rpmerr_a < 0.0 ]
    (junction 42) -> (junction 44) [order 2]
    (junction 44) -> (junction 48) [order 2] : { ml_iscpsi_sw = 1; }
    (junction 44) -> (junction 46) [order 1] : [ rpmerr_a >= 0.0 ]
    (junction 45) -> (junction 49) [order 1] : [ (ETC_HP == 1) && ...
        |   (etc_des_ta <= ETC_CL_TP) ]
    (junction 45) -> (junction 49) [order 2] : [ (ETC_HP == 0) && ...
        |   (iac_at_lolm == 1) ]
    (junction 46) -> (junction 50) : [ (iac_at_hilm == 1) ||...
        |   (iac_fb_satx == 1) ]
    (junction 48) -> (junction 51) [order 1] : [ rpmerr_a > 0.0 ]
        | {ml_tc_sw = 2; }
    (junction 48) -> (junction 51) [order 2] : {ml_tc_sw = 1; }
    (junction 49) -> (junction 50)
    (junction 50) -> (junction 53) : { ml_iscpsi_sw = 2; }
    (junction 51) -> (junction 53)
    (junction 53) -> (junction 54) : { do_iscpsi_calc; }
    (junction 54) -> (junction 57) [order 1] : [ runuptmr < ISC_MAN_TM ]
        | { ml_prop_sw = 2; }
    (junction 54) -> (junction 55) [order 2] : { do_fn852a_calc;
        |   ml_prop_sw = 1; }
    (junction 55) -> (junction 56) [order 2] : /* TCPRO_LT */
        | { ml_tcpro_sw = 2; }
    (junction 55) -> (junction 56) [order 1] : /* TCPRO_GT */
        | [ isc_a_prop_tmp > isc_a_prop ]
        | { ml_tcpro_sw = 1; }
    (junction 56) -> (junction 57)
    (junction 57) -> (junction 58) [order 1] : /* Filtered RPMERR calculation, used for deriviative air control term */
        | [  (dsdrpm == dsdrpm_lst) ...
        |  && ( engine_speed < (dsdrpm + DSDRPM_OFF)) ]
        | { ml_der_sw = 2; }
    (junction 57) -> (junction 58) [order 2] : { ml_der_sw = 1;  }
    (junction 58) -> (junction 59) [order 2]
    (junction 58) -> (junction 59) [order 1] : [   (powsfg == 0)...
        |  || ( (ipsibr + iscpsi) >= PSIBRN_PS)...
        |  || (iscpsi >= 0.0) ]
        | { do_ipsibr_calc; }
    (junction 59) -> (junction 60) : {do_idle_ppm_calc; }
  state idle_rpm_controller [parallel]
    settings: executionOrder=3
    idle_rpm_controller -> (junction 47)
    (default) -> (junction 47)
    (junction 47) -> (junction 52) [order 1] : [ ml_irpm_init_flg == 1 ]
        | { ml_init_sw = 2;
        |   idle_rpm_controller_initialisation.trig; }
    (junction 47) -> (junction 52) [order 2] : { ml_init_sw = 1;
        |   normal_rpm_control.trig; }
  data: iac_fb_satx output boolean size=1; iac_at_hilm input boolean size=1; iac_at_lolm input boolean size=1; powsfg input boolean size=1; PSIBRM parameter double size=1; PSIBRN_PS parameter double size=1; ml_irpm_init_flg input boolean size=1; etc_des_ta input single size=1; ETC_CL_TP parameter single size=1; dsdrpm_lst input single size=1; runuptmr input single size=1; ml_tc_sw output int8 size=1; ml_prop_sw output int8 size=1; ml_tcpro_sw output uint8 size=1; ml_der_sw output int8 size=1; ETC_HP parameter boolean size=1; ml_init_sw output int8 size=1 =1; rpmerr_a input double size=1; engine_speed input uint8 size=1; dsdrpm input single size=1; ipsibr input double size=1; iscpsi input double size=1; isc_a_prop input single size=1; isc_a_prop_tmp input single size=1; ISC_MAN_TM parameter single size=1; ml_iscpsi_sw output int8 size=1; DSDRPM_OFF parameter single size=1
  events: trig local EITHER_EDGE_EVENT; trig local EITHER_EDGE_EVENT; trig_idle_rpm_controller input FUNCTION_CALL_EVENT; do_iscpsi_calc output FUNCTION_CALL_EVENT; do_idle_ppm_calc output FUNCTION_CALL_EVENT; do_rpmerr_calc output FUNCTION_CALL_EVENT; do_ipsibr_calc output FUNCTION_CALL_EVENT; do_fn852a_calc output FUNCTION_CALL_EVENT

== stateflow chart mfordmodel_v1/iac_v04_001_001/iac_executive/misc_calcs/osc_response_logic_ctl ==
  (default) -> (junction 13) : trig_osc_response_logic
  (junction 13) -> (junction 18) [order 1] : /* no substitution request */
      | [subst_req_0 == 0]
  (junction 13) -> (junction 14) [order 2]
  (junction 14) -> (junction 18) [order 5]
  (junction 14) -> (junction 17) [order 1] : [crkflg==1 &&...
      |  tslpip < 2.0]
  (junction 14) -> (junction 15) [order 4] : [runup_flg == 0]
  (junction 14) -> (junction 17) [order 3] : [mfmflg == 1 ...
      | && tfmflg ==1]
  (junction 14) -> (junction 17) [order 2] : [er_isc_hld == 1]
  (junction 15) -> (junction 16) [order 2] : [crkflg == 0]
  (junction 15) -> (junction 16) [order 1] : [tslpip < 2.0]
  (junction 16) -> (junction 17)
  (junction 17) -> (junction 18) : {
      | do_osc_response ;
      | }
  data: runup_flg input boolean size=1; crkflg input boolean size=1; er_isc_hld input boolean size=1; mfmflg input boolean size=1; subst_req_0 input boolean size=1; tfmflg input boolean size=1; tslpip input double size=1
  events: do_osc_response output FUNCTION_CALL_EVENT; trig_osc_response_logic input FUNCTION_CALL_EVENT

== stateflow chart mfordmodel_v1/iac_v04_001_001/activate_desired_rpm/activate_desired_rpm_ctl ==
  (default) -> (junction 23) : trig_activate_desired_rpm
  (junction 23) -> (junction 24) [order 1] : /* trans_oil_temp_rpm_request() */
      | [ pdl == REVERSE ]
      | { ml_tot_sw = 1; }
  (junction 23) -> (junction 24) [order 2] : { ml_tot_sw = 2; }
  (junction 24) -> (junction 25) [order 1] : /* extended_idle_rpm_request() */
      | [     (dndsup == 0)...
      |  && (tfmflg == 0) ]
      | { ml_xtend_sw = 1; }
  (junction 24) -> (junction 25) [order 2] : { ml_xtend_sw = 2; }
  (junction 25) -> (junction 26) : {  trig_rpm_adders_fans_and_pw_steer; }
      |
      | /* trans_spin_loss_rpm_request() */
  (junction 26) -> (junction 28) [order 1] : [ TRLOAD < 6 ]
      | { ml_tsl_sw = 1; }
  (junction 26) -> (junction 27) [order 2]
  (junction 27) -> (junction 28) [order 2] : { ml_tsl_sw = 1; }
  (junction 27) -> (junction 28) [order 1] : [    (vsfmflg == 0)...
      |  && (pdl == NEUTRAL)...
      |  && (pdl_error == 0)...
      |  && (tfmflg == 0)...
      |  && (tsfmflg == 0) ]
      | { ml_tsl_sw = 2; }
  (junction 28) -> (junction 29) [order 1] : /* iac_inferred_ambient_temp() */
      |
      | [     (afmflg == 0)...
      |  && (cfmflg == 0)...
      |  && (vsfmflg == 0) ]
      | { ml_inf_amb_sw = 1; }
  (junction 28) -> (junction 29) [order 2] : { ml_inf_amb_sw = 2; }
  (junction 29) -> (junction 30) : { do_inf_amb_calc; }
      |
      | /* air_conditioning_rpm_request() */
  (junction 30) -> (junction 32) [order 1] : [ acrqst == 1]
      | { ac_rpm_flg = 1; }
  (junction 30) -> (junction 31) [order 2]
  (junction 31) -> (junction 32) [order 1] : [ aciotmr > AC_OFF_DLY ]
      | { ac_rpm_flg = 0; }
  (junction 31) -> (junction 32) [order 2]
  (junction 32) -> (junction 34) [order 2] : { ml_ac_sw = 3; }
  (junction 32) -> (junction 33) [order 1] : [ ac_rpm_flg == 1]
  (junction 33) -> (junction 34) [order 1] : [ (dndsup == 0)...
      |  || ( AUTO_TRNS_SW == 0) ]
      | { ml_ac_sw = 1; }
  (junction 33) -> (junction 34) [order 2] : { ml_ac_sw = 2; }
  (junction 34) -> (junction 35) : { do_rpm_calcs;
      |   trig_hicam_rpm_request;
      |   trig_base_rpm_and_select_logic; }
  data: ml_tot_sw output uint8 size=1; ml_xtend_sw output uint8 size=1; ml_tsl_sw output uint8 size=1; ml_inf_amb_sw output uint8 size=1; pdl input uint8 size=1; REVERSE constant uint8 size=1 =60; pdl_error input boolean size=1; tfmflg input boolean size=1; vsfmflg input boolean size=1; NEUTRAL constant uint8 size=1 =50; tsfmflg input boolean size=1; TRLOAD parameter uint8 size=1; afmflg input boolean size=1; cfmflg input boolean size=1; acrqst input boolean size=1; aciotmr input double size=1; dndsup input boolean size=1; AUTO_TRNS_SW parameter uint8 size=1; ml_ac_sw output uint8 size=1; ac_rpm_flg local boolean size=1; AC_OFF_DLY parameter double size=1
  events: trig_activate_desired_rpm input FUNCTION_CALL_EVENT; do_inf_amb_calc output FUNCTION_CALL_EVENT; trig_rpm_adders_fans_and_pw_steer output FUNCTION_CALL_EVENT; do_rpm_calcs output FUNCTION_CALL_EVENT; trig_hicam_rpm_request output FUNCTION_CALL_EVENT; trig_base_rpm_and_select_logic output FUNCTION_CALL_EVENT

== stateflow chart mfordmodel_v1/iac_v04_001_001/iac_executive/fault_code_setting/TIMER_DT_in/Timer Control ==
  state TIMER_control
    state CHANGE_timer
      /* only one
      flag active */
      CHANGE_timer -> (junction 25) [order 1]
      (junction 26) -> (junction 25) [order 2]
      (junction 25) -> (junction 28) [order 1] : [incr_flag==1]
          | {
          | count_direction=1;
          | }
      (junction 25) -> (junction 28) [order 2] : [decr_flag==1]
          | {
          | count_direction= -1;
          | }
      (default) -> (junction 26)
      (junction 26) -> (junction 30) [order 1] : [reset_flag == 1]
          | {reset_flag = 0;}
      (junction 28) -> (junction 30) : {
          | do_delta_time;
          | do_timer;
          | }
    state HOLD_timer
      /* flags both
      active or both
      inactive */
      (default) -> (junction 27)
      (junction 27) -> (junction 29) : {
          | count_direction=0;
          | do_delta_time;
          | }
    (default) -> (junction 23)
    (junction 23) -> HOLD_timer [order 2]
    (junction 23) -> CHANGE_timer [order 1] : [incr_flag!=decr_flag]
    HOLD_timer -> (junction 27) [order 2]
    HOLD_timer -> CHANGE_timer [order 1] : [incr_flag!=decr_flag]
    CHANGE_timer -> HOLD_timer [order 1] : [incr_flag==decr_flag]
  (default) -> (junction 24)
  (junction 24) -> TIMER_control [order 2]
  (junction 24) -> TIMER_control [order 1] : trig_reset
      | {
      | reset_flag=1;
      | do_delta_time;
      | do_timer;
      | }
  TIMER_control -> TIMER_control : trig_reset
      | {
      | reset_flag=1;
      | do_delta_time;
      | do_timer;
      | }
  data: count_direction output int16; incr_flag input boolean; decr_flag input boolean; reset_flag output boolean [0..1]
  events: do_delta_time output FUNCTION_CALL_EVENT; do_timer output FUNCTION_CALL_EVENT; trig_timer input FUNCTION_CALL_EVENT; trig_reset input FUNCTION_CALL_EVENT

== stateflow chart mfordmodel_v1/iac_v04_001_001/normal_mode/iscflg_module/preposition/preposition_ctl ==
  (default) -> (junction 5)
  (junction 5) -> (junction 6) [order 2] : {
      | ml_mul_sw = 1;
      | }
  (junction 5) -> (junction 6) [order 1] : [ dndsup == 1 ]
      | {
      | ml_mul_sw = 2;
      | }
  (junction 6) -> (junction 7) : {
      | do_idle_ppm_calc;
      | trig_das_min_clip_prepos;
      | }
  data: dndsup input boolean size=1; ml_mul_sw output uint8 size=1
  events: trig_das_min_clip_prepos output FUNCTION_CALL_EVENT; do_idle_ppm_calc output FUNCTION_CALL_EVENT; trig_preposition input FUNCTION_CALL_EVENT

== stateflow chart mfordmodel_v1/iac_v04_001_001/activate_desired_rpm/base_rpm_and_select_logic/base_rpm_and_select_logic_ctl ==
  state dsdrpm_max10 [parallel]
    settings: executionOrder=1
    dsdrpm_max10 -> (junction 49) : trig
    (default) -> (junction 49) : trig
    (junction 49) -> (junction 51) [order 1] : [is_tot_rpm > is_base_rpm]
        | { dsdrpm_tmp = is_tot_rpm;
        |    is_source = IS_SOURCE_TOT_RPM; }
    (junction 49) -> (junction 51) [order 2] : { dsdrpm_tmp = is_base_rpm; }
    (junction 51) -> (junction 54) [order 1] : [is_xtend_rpm > dsdrpm_tmp]
        | { dsdrpm_tmp = is_xtend_rpm;
        |   is_source = IS_SOURCE_XTEND_RPM; }
    (junction 51) -> (junction 54) [order 2]
    (junction 54) -> (junction 56) [order 1] : [is_ps_rpm > dsdrpm_tmp]
        | { dsdrpm_tmp = is_ps_rpm;
        |   is_source = IS_SOURCE_PS_RPM; }
    (junction 54) -> (junction 56) [order 2]
    (junction 56) -> (junction 59) [order 2]
    (junction 56) -> (junction 59) [order 1] : [is_ac_rpm > dsdrpm_tmp]
        | { dsdrpm_tmp = is_ac_rpm;
        |   is_source = IS_SOURCE_AC_RPM; }
    (junction 59) -> (junction 61) [order 1] : [is_alt_rpm > dsdrpm_tmp]
        | { dsdrpm_tmp = is_alt_rpm;
        |   is_source = IS_SOURCE_ALT_RPM; }
    (junction 59) -> (junction 61) [order 2]
    (junction 61) -> (junction 63) [order 2]
    (junction 61) -> (junction 63) [order 1] : [is_tsl_rpm > dsdrpm_tmp]
        | { dsdrpm_tmp = is_tsl_rpm;
        |   is_source = IS_SOURCE_TSL_RPM; }
    (junction 63) -> (junction 65) [order 2]
    (junction 63) -> (junction 65) [order 1] : [is_hedf_rpm > dsdrpm_tmp]
        | { dsdrpm_tmp = is_hedf_rpm;
        |   is_source = IS_SOURCE_HEDF_RPM; }
    (junction 65) -> (junction 67) [order 1] : [is_heater_core_rpm_tmp > dsdrpm_tmp]
        | { dsdrpm_tmp = is_heater_core_rpm_tmp;
        |   is_source = IS_SOURCE_HEATER_CORE_RPM; }
    (junction 65) -> (junction 67) [order 2]
  state MAIN [parallel]
    settings: executionOrder=2
    MAIN -> (junction 50) : trig_base_rpm_and_select_logic
    (default) -> (junction 50) : trig_base_rpm_and_select_logic
    (junction 50) -> (junction 52) [order 1] : [   ( AUTO_TRNS_SW == 0)...
        |  || (dndsup == 0) ]
        | { auto_or_neutral_tmp = 1; }
    (junction 50) -> (junction 52) [order 2] : { auto_or_neutral_tmp = 0; }
    (junction 52) -> (junction 55) [order 1] : [ alt_cal_flg == 1 ]
    (junction 52) -> (junction 53) [order 2]
    (junction 53) -> (junction 62) [order 1] : [ cool_flg == 1 ]
        | { is_base_rpm = COOL_BASE;
        |   is_source =...
        |   IS_SOURCE_RPM_BASE_FAILSAFE_COOLING; }
    (junction 53) -> (junction 57) [order 2]
    (junction 55) -> (junction 58) [order 2] : {  is_base_rpm =...
        | IS_DRBASE_A__A; }
    (junction 55) -> (junction 58) [order 1] : [ auto_or_neutral_tmp == 1]
        | { is_base_rpm =...
        |  IS_NUBASE_A__A; }
    (junction 57) -> (junction 60) [order 2] : {  is_base_rpm =...
        |    IS_DRBASE__A; }
    (junction 57) -> (junction 60) [order 1] : [ auto_or_neutral_tmp == 1]
        | { is_base_rpm =...
        |  IS_NUBASE__A; }
    (junction 58) -> (junction 62) : { is_source =...
        |   IS_SOURCE_RPM_BASE_ANTI_PLUG_FOUL; }
    (junction 60) -> (junction 62) : { is_source =...
        |   IS_SOURCE_RPM_BASE_NEUTRAL_DRIVE; }
    (junction 62) -> (junction 64) : { is_base_rpm += hicam; }
    (junction 64) -> (junction 66) [order 1] : [ auto_or_neutral_tmp == 1]
        | { ml_htr_core_calc_sw = 1;
        |  do_htr_core_rpm_calc; }
    (junction 64) -> (junction 66) [order 2] : { ml_htr_core_calc_sw = 2;
        |   do_htr_core_rpm_calc; }
    (junction 66) -> (junction 68) [order 2] : { dsdrpm_max10.trig; }
    (junction 66) -> (junction 68) [order 1] : [ er_isc_req == 1]
        | { dsdrpm_tmp = er_rpm;
        |   is_source = IS_SOURCE_ER_RPM; }
    (junction 68) -> (junction 69) [order 1] : [ alt_cal_flg == 1]
        | { is_gpas_clip = ISCLPD_ALT; }
    (junction 68) -> (junction 69) [order 2] : { is_gpas_clip = ISCLPD; }
    (junction 69) -> (junction 70) [order 1] : /* dsdrpm2()   */
        | [   ( auto_or_neutral_tmp == 0) ...
        |   && ( is_gpas_clip < dsdrpm_tmp) ]
        | { dsdrpm_tmp = is_gpas_clip;
        |    is_source = IS_SOURCE_GPAS_MIN_CLIP; }
    (junction 69) -> (junction 70) [order 2]
    (junction 70) -> (junction 71) [order 2]
    (junction 70) -> (junction 72) [order 1] : [ runup_flg == 0 ]
        | { dsdrpm_tc_tmp = 0.0; }
    (junction 71) -> (junction 72) [order 2] : { dsdrpm_tc_tmp = DSDRPM_DN_TC; }
    (junction 71) -> (junction 72) [order 1] : [ dsdrpm_tmp > dsdrpm_lst ]
        | { dsdrpm_tc_tmp = DSDRPM_UP_TC; }
    (junction 72) -> (junction 73) : { do_dsdrpm_calc; }
  data: is_source output uint8 size=1; dsdrpm_tmp output double size=1; dsdrpm_tc_tmp output double size=1; ml_htr_core_calc_sw output uint8 size=1; is_tot_rpm input double size=1; IS_SOURCE_TOT_RPM constant uint8 size=1 =7; is_xtend_rpm input double size=1; IS_SOURCE_XTEND_RPM constant uint8 size=1 =6; is_ps_rpm input double size=1; IS_SOURCE_PS_RPM constant uint8 size=1 =10; is_ac_rpm input double size=1; IS_SOURCE_AC_RPM constant uint8 size=1 =2; is_alt_rpm input double size=1; IS_SOURCE_ALT_RPM constant uint8 size=1 =5; is_tsl_rpm input double size=1; IS_SOURCE_TSL_RPM constant uint8 size=1 =9; is_hedf_rpm input double size=1; IS_SOURCE_HEDF_RPM constant uint8 size=1 =11; IS_SOURCE_HEATER_CORE_RPM constant uint8 size=1 =12; er_rpm input double size=1; hicam input double size=1; dndsup input boolean size=1; auto_or_neutral_tmp local boolean size=1; alt_cal_flg input boolean size=1; IS_DRBASE__A parameter double size=1; IS_NUBASE__A parameter double size=1; IS_DRBASE_A__A parameter double size=1; IS_NUBASE_A__A parameter double size=1; cool_flg input boolean size=1; IS_SOURCE_RPM_BASE_ANTI_PLUG_FOUL constant uint8 size=1 =22; IS_SOURCE_ER_RPM constant uint8 size=1 =1; IS_SOURCE_GPAS_MIN_CLIP constant uint8 size=1; DSDRPM_DN_TC parameter double size=1; DSDRPM_UP_TC parameter double size=1; runup_flg input boolean size=1; dsdrpm_lst input double size=1; er_isc_req input boolean size=1; is_heater_core_rpm_tmp input double size=1; is_gpas_clip local double size=1; COOL_BASE parameter double size=1; AUTO_TRNS_SW parameter uint8 size=1; is_base_rpm local double size=1; ISCLPD parameter double size=1; ISCLPD_ALT parameter double size=1; IS_SOURCE_RPM_BASE_FAILSAFE_COOLING constant uint8 size=1 =21; IS_SOURCE_RPM_BASE_NEUTRAL_DRIVE constant uint8 size=1 =20
  events: trig local EITHER_EDGE_EVENT; trig_base_rpm_and_select_logic input FUNCTION_CALL_EVENT; do_dsdrpm_calc output FUNCTION_CALL_EVENT; do_htr_core_rpm_calc output FUNCTION_CALL_EVENT
